simulink model "kalman_filter"  (R2024b)
settings: Solver=FixedStepAuto  StartTime=0.0  StopTime=10.0  FixedStep=0.01  RelTol=1e-3
settings Model: Creator=ARULPAVALAN S A  LastModifiedBy=ARULPAVALAN S A

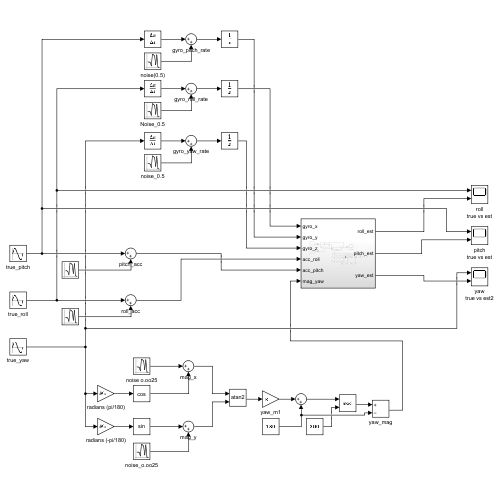
[thumbnail: Simulink's stored preview of the top-level diagram]
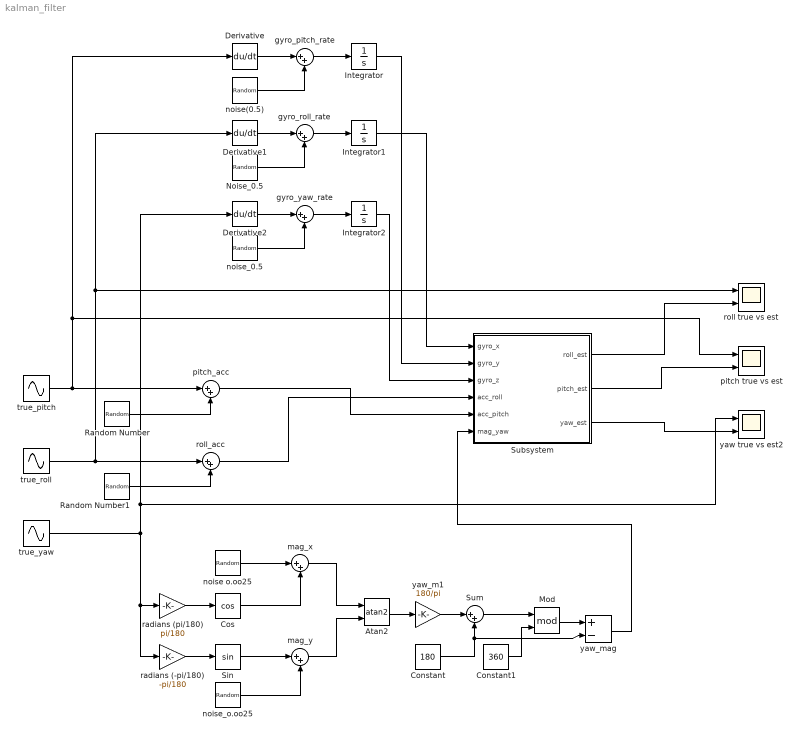
== system kalman_filter ==
  Atan2 : Trigonometry  Operator=atan2
  Constant : Constant  Value=180
  Constant1 : Constant  Value=360
  Cos : Trigonometry  Operator=cos
  Derivative : Derivative
  Derivative1 : Derivative
  Derivative2 : Derivative
  Integrator : Integrator
  Integrator1 : Integrator
  Integrator2 : Integrator
  Mod : Math  Operator=mod
  Noise_0.5 : RandomNumber  Variance=0.25  SampleTime=0.1
  Random Number : RandomNumber  Variance=2.25  SampleTime=0.1
  Random Number1 : RandomNumber  Variance=2.25  SampleTime=0.1
  Sin : Trigonometry
  Subsystem : Subsystem
  Sum : Sum  Inputs=|++
  "gyro_pitch_rate " : Sum  Inputs=|++
  "gyro_roll_rate " : Sum  Inputs=|++
  "gyro_yaw_rate " : Sum  Inputs=|++
  mag_x : Sum  Inputs=|++
  mag_y : Sum  Inputs=|++
  noise o.oo25 : RandomNumber  Variance=0.0025  SampleTime=0.1
  noise(0.5) : RandomNumber  Variance=0.25  SampleTime=0.1
  noise_0.5 : RandomNumber  Variance=0.25  SampleTime=0.1
  noise_o.oo25 : RandomNumber  Variance=0.0025  SampleTime=0.1
  pitch true vs est : Scope  NumInputPorts=2
  pitch_acc : Sum  Inputs=|++
  radians (-pi/180) : Gain  Gain=-pi/180
  radians (pi/180) : Gain  Gain=pi/180
  roll true vs est : Scope  NumInputPorts=2
  roll_acc : Sum  Inputs=|++
  true_pitch : Sin  Amplitude=3  Frequency=0.6283  SampleTime=0
  true_roll : Sin  Amplitude=5  Frequency=0.6283  SampleTime=0
  true_yaw : Sin  Amplitude=10  Frequency=0.6283  SampleTime=0
  yaw true vs est2 : Scope  NumInputPorts=2
  yaw_m1 : Gain  Gain=180/pi
  yaw_mag : Sum  Inputs=+-
  wires:
  "gyro_roll_rate "/1 -> Integrator1/1
  noise(0.5)/1 -> "gyro_pitch_rate "/2
  Noise_0.5/1 -> "gyro_roll_rate "/2
  "gyro_yaw_rate "/1 -> Integrator2/1
  Derivative/1 -> "gyro_pitch_rate "/1
  Derivative2/1 -> "gyro_yaw_rate "/1
  "gyro_pitch_rate "/1 -> Integrator/1
  noise_0.5/1 -> "gyro_yaw_rate "/2
  Derivative1/1 -> "gyro_roll_rate "/1
  true_roll/1 -> roll_acc/1, roll true vs est/1, Derivative1/1
  true_pitch/1 -> pitch_acc/1, pitch true vs est/1, Derivative/1
  Random Number/1 -> pitch_acc/2
  Random Number1/1 -> roll_acc/2
  Mod/1 -> yaw_mag/1
  yaw_m1/1 -> Sum/1
  Constant/1 -> Sum/2, yaw_mag/2
  Constant1/1 -> Mod/2
  Sum/1 -> Mod/1
  noise_o.oo25/1 -> mag_y/2
  mag_y/1 -> Atan2/2
  radians (-pi/180)/1 -> Sin/1
  mag_x/1 -> Atan2/1
  Cos/1 -> mag_x/2
  noise o.oo25/1 -> mag_x/1
  true_yaw/1 -> yaw true vs est2/1, Derivative2/1, radians (-pi/180)/1, radians (pi/180)/1
  Sin/1 -> mag_y/1
  radians (pi/180)/1 -> Cos/1
  Atan2/1 -> yaw_m1/1
  pitch_acc/1 -> Subsystem/5(acc_pitch)
  roll_acc/1 -> Subsystem/4(acc_roll)
  yaw_mag/1 -> Subsystem/6(mag_yaw)
  Integrator1/1 -> Subsystem/1(gyro_x)
  Integrator/1 -> Subsystem/2(gyro_y)
  Integrator2/1 -> Subsystem/3(gyro_z)
  Subsystem/1(roll_est) -> roll true vs est/2
  Subsystem/2(pitch_est) -> pitch true vs est/2
  Subsystem/3(yaw_est) -> yaw true vs est2/2

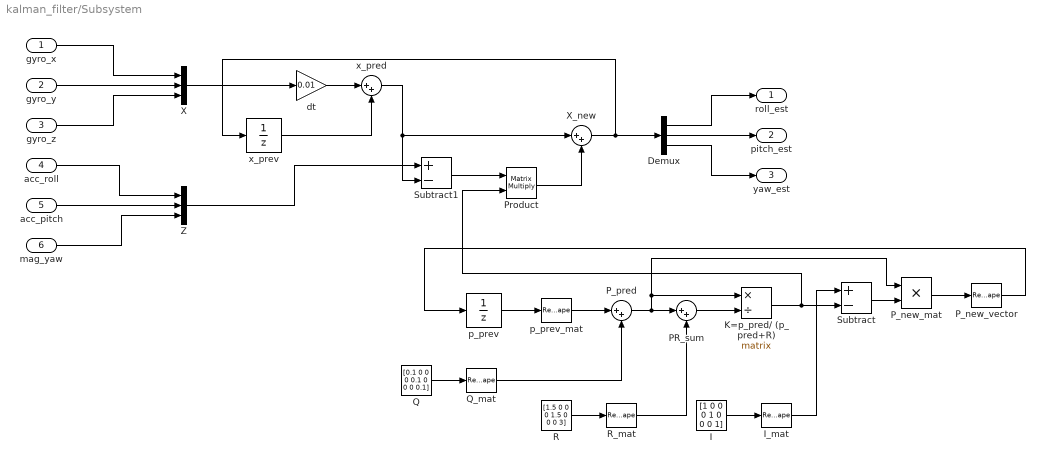
== system kalman_filter/Subsystem ==
  gyro_x : Inport
  gyro_y : Inport  Port=2
  gyro_z : Inport  Port=3
  acc_roll : Inport  Port=4
  acc_pitch : Inport  Port=5
  mag_yaw : Inport  Port=6
  Demux : Demux  Outputs=3
  I : Constant  Value=[1 0 0 0 1 0 0 0 1]
  I_mat : Reshape  OutputDimensionality=Customize  OutputDimensions=[3,3]
  K=p_pred/ (p_pred+R) : Product  Inputs=*/  Multiplication=Matrix(*)
  "PR_sum " : Sum  Inputs=|++
  P_new_mat : Product
  P_new_vector : Reshape  OutputDimensionality=Customize  OutputDimensions=[1,9]
  "P_pred " : Sum  Inputs=|++
  Product : Product  Multiplication=Matrix(*)
  Q : Constant  Value=[0.1 0 0 0 0.1 0 0 0 0.1]
  Q_mat : Reshape  OutputDimensionality=Customize  OutputDimensions=[3,3]
  R : Constant  Value=[1.5 0 0 0 1.5 0 0 0 3]
  R_mat : Reshape  OutputDimensionality=Customize  OutputDimensions=[3,3]
  Subtract : Sum  Inputs=+-
  Subtract1 : Sum  Inputs=+-
  X : Mux  Inputs=3
  X_new : Sum  Inputs=|++
  Z : Mux  Inputs=3
  dt : Gain  Gain=0.01
  p_prev : UnitDelay  InitialCondition=[1 0 0 0 1 0 0 0 1]  SampleTime=-1  HasFrameUpgradeWarning=on
  p_prev_mat : Reshape  OutputDimensionality=Customize  OutputDimensions=[3,3]
  "x_pred " : Sum  Inputs=|++
  x_prev : UnitDelay  SampleTime=-1  HasFrameUpgradeWarning=on
  roll_est : Outport
  pitch_est : Outport  Port=2
  yaw_est : Outport  Port=3
  wires:
  R_mat/1 -> "PR_sum "/2
  Subtract/1 -> P_new_mat/2
  X_new/1 -> Demux/1, x_prev/1
  "PR_sum "/1 -> K=p_pred/ (p_pred+R)/2
  K=p_pred/ (p_pred+R)/1 -> Product/2, Subtract/2
  "P_pred "/1 -> P_new_mat/1, K=p_pred/ (p_pred+R)/1, "PR_sum "/1
  R/1 -> R_mat/1
  X/1 -> dt/1
  mag_yaw/1 -> Z/3
  "x_pred "/1 -> X_new/1, Subtract1/2
  P_new_mat/1 -> P_new_vector/1
  acc_roll/1 -> Z/1
  Q/1 -> Q_mat/1
  Subtract1/1 -> Product/1
  Demux/1 -> roll_est/1
  Demux/3 -> yaw_est/1
  Q_mat/1 -> "P_pred "/2
  I_mat/1 -> Subtract/1
  gyro_z/1 -> X/3
  p_prev/1 -> p_prev_mat/1
  p_prev_mat/1 -> "P_pred "/1
  Product/1 -> X_new/2
  x_prev/1 -> "x_pred "/2
  dt/1 -> "x_pred "/1
  gyro_x/1 -> X/1
  P_new_vector/1 -> p_prev/1
  Demux/2 -> pitch_est/1
  I/1 -> I_mat/1
  acc_pitch/1 -> Z/2
  gyro_y/1 -> X/2
  Z/1 -> Subtract1/1
